simulink model "gyro"  (R2018b)
settings: Solver=VariableStepAuto  StartTime=0.0  StopTime=1  RelTol=1e-3
libraries: dspspect3 x2, simulink x1
settings Model: Creator=dongdaming  LastModifiedBy=dongdaming

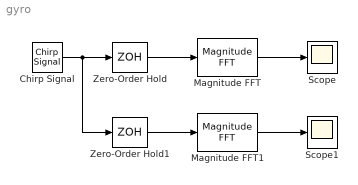
== system gyro ==
  Chirp Signal : simulink/Sources/Chirp Signal  f1=0.1  T=100  f2=0.0001
  Magnitude FFT : dspspect3/Magnitude FFT  mag_or_magsq=Magnitude squared  FFTImplementation=Auto  fftLenInherit=off  fftsize=256  WrapInput=on
      settings: SourceProductName=DSP System Toolbox  SourceProductBaseCode=DS
  Magnitude FFT1 : dspspect3/Magnitude FFT  mag_or_magsq=Magnitude squared  FFTImplementation=Auto  fftLenInherit=off  fftsize=256  WrapInput=on
      settings: SourceProductName=DSP System Toolbox  SourceProductBaseCode=DS
  Scope : Scope
  Scope1 : Scope
  Zero-Order Hold : ZeroOrderHold  SampleTime=0.002
  Zero-Order Hold1 : ZeroOrderHold  SampleTime=0.0002
  wires:
  Zero-Order Hold/1 -> Magnitude FFT/1
  Chirp Signal/1 -> Zero-Order Hold1/1, Zero-Order Hold/1
  Zero-Order Hold1/1 -> Magnitude FFT1/1
  Magnitude FFT/1 -> Scope/1
  Magnitude FFT1/1 -> Scope1/1
